simulink model "DYpid"  (R2018b)
settings: Solver=ode4  StartTime=0.0  StopTime=100  FixedStep=0.1  RelTol=1e-3
libraries: simulink x1
settings Model: Creator=15486  LastModifiedBy=麦克飘
settings SFSimCC: SimUseLocalCustomCode=off
settings RTWCC: RTWUseLocalCustomCode=off
settings CodeAppCC: StateflowObjectComments=on

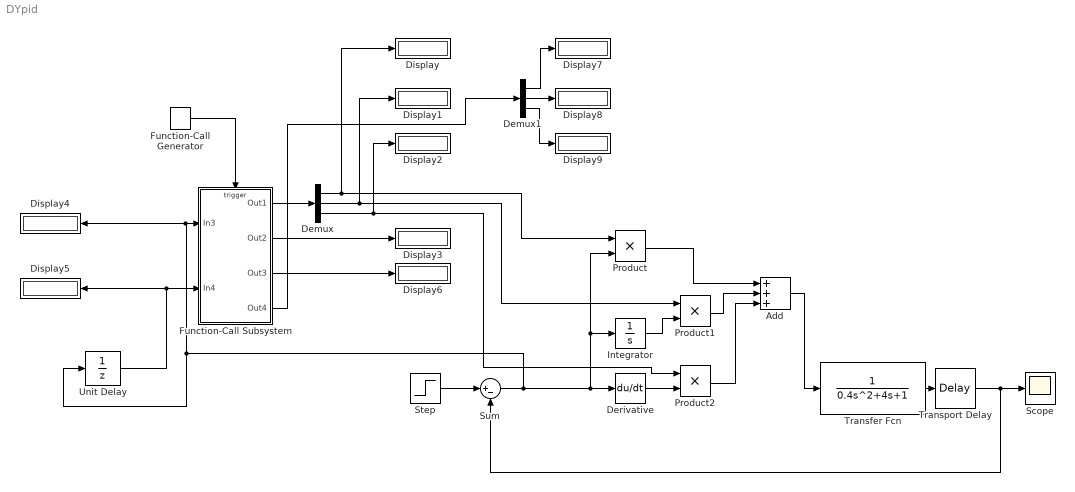
== system DYpid ==
  Add : Sum  Inputs=+++
  Demux : Demux  Outputs=3
  Demux1 : Demux  Outputs=3
  Derivative : Derivative
  Display{,1..9} (10 alike) : Display
  Function-Call Generator : simulink/Ports & Subsystems/Function-Call Generator  sample_time=0.1  numberOfIterations=1
  Function-Call Subsystem : Subsystem  TreatAsAtomicUnit=on
  Integrator : Integrator
  Product : Product
  Product1 : Product
  Product2 : Product
  Scope : Scope
  Step : Step  Time=0  After=10  SampleTime=0
  Sum : Sum  Inputs=|+-
  Transfer Fcn : TransferFcn  Numerator=1  Denominator=[0.4 4 1]
  Transport Delay : TransportDelay  DelayTime=2
  Unit Delay : UnitDelay  SampleTime=-1
  wires:
  Transfer Fcn/1 -> Transport Delay/1
  Sum/1 -> Display4/1, Function-Call Subsystem/1(In3), Unit Delay/1, Derivative/1, Product/2, Integrator/1
  Step/1 -> Sum/1
  Transport Delay/1 -> Sum/2, Scope/1
  Demux/2 -> Display1/1, Product1/1
  Product/1 -> Add/1
  Product1/1 -> Add/2
  Add/1 -> Transfer Fcn/1
  Product2/1 -> Add/3
  Integrator/1 -> Product1/2
  Derivative/1 -> Product2/2
  Demux/3 -> Display2/1, Product2/1
  Function-Call Subsystem/1(Out1) -> Demux/1
  Function-Call Subsystem/4(Out4) -> Demux1/1
  Demux/1 -> Display/1, Product/1
  Function-Call Subsystem/2(Out2) -> Display3/1
  Unit Delay/1 -> Display5/1, Function-Call Subsystem/2(In4)
  Function-Call Generator/1 -> Function-Call Subsystem/Trigger
  Function-Call Subsystem/3(Out3) -> Display6/1
  Demux1/1 -> Display7/1
  Demux1/3 -> Display9/1
  Demux1/2 -> Display8/1

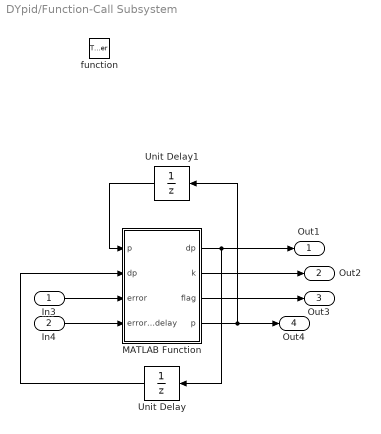
== system DYpid/Function-Call Subsystem ==
  In3 : Inport
  In4 : Inport  Port=2
  function : TriggerPort  TriggerType=function-call  VariantControl=Variant
  MATLAB Function : MATLAB Function  TreatAsAtomicUnit=on
  Unit Delay : UnitDelay  SampleTime=-1
  Unit Delay1 : UnitDelay  SampleTime=-1
  Out1 : Outport
  Out2 : Outport  Port=2
  Out3 : Outport  Port=3
  Out4 : Outport  Port=4
  wires:
  MATLAB Function/1(dp) -> Unit Delay/1, Out1/1
  MATLAB Function/2(k) -> Out2/1
  In3/1 -> MATLAB Function/3(error)
  In4/1 -> MATLAB Function/4(error_delay)
  MATLAB Function/3(flag) -> Out3/1
  MATLAB Function/4(p) -> Unit Delay1/1, Out4/1
  Unit Delay1/1 -> MATLAB Function/1("p ")
  Unit Delay/1 -> MATLAB Function/2("dp ")

== matlab function DYpid/Function-Call Subsystem/MATLAB Function ==
  data: p input; dp input; dp output; error input; error_delay input; k output; flag output; p output
function [dp,k,flag,p]  = fcn( p,dp,error,error_delay)
error = abs(error);
error_delay = abs(error_delay);

tol = 0.2;
condi = 1;
flag =0;
k = 0;
% persistent k;
% if isempty(k)
%    k = 0;
% end



%  while condi ==1


     for i = 1:3
         p(i)= p(i)+ dp(i);
         if error < error_delay
             flag = 1;
             error_delay = error;
             dp(i) = dp(i)*1.1;
            
         else
             p(i) = p(i) - 2*dp(i);
             if error < error_delay
                 flag =2;
             error_delay = error;
             dp(i) = 1.1* dp(i);
             else
                 p(i) = p(i)+dp(i);
                 flag =3;
                 dp(i) = dp(i)*0.9;
             end
         end
     end
     k = k+1;
%      if k ==10
% %      if sum(dp)<=0.1;
%          condi = 2;
%         
%      end
     
%  end
        
end
